simulink model "testing_embedded_matlab_functions"  (Simulink 7.5)
settings: Solver=ode45  StartTime=0.0  StopTime=10.0  RelTol=1e-3
settings Model: Creator=konstantinos  LastModifiedBy=konstantinos

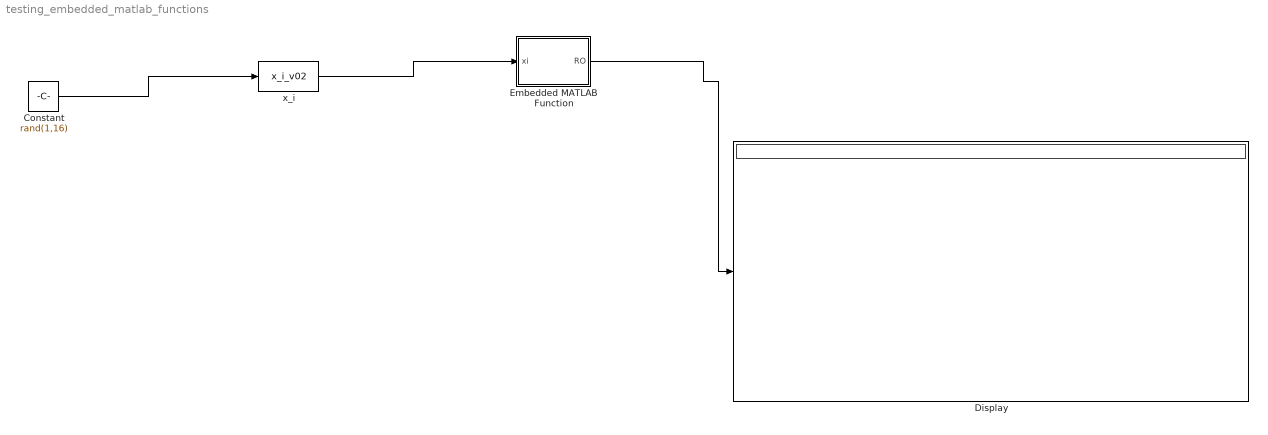
== system testing_embedded_matlab_functions ==
  Constant : Constant  Value=rand(1,16)  OutDataType=fixdt(1, 16)  OutScaling=2^0
  Display : Display
  Embedded MATLAB Function : Stateflow chart  TreatAsAtomicUnit=on
  x_i : MATLABFcn  MATLABFcn=x_i_v02  Output1D=off
  wires:
  Embedded MATLAB Function/1(RO) -> Display/1
  Constant/1 -> x_i/1
  x_i/1 -> Embedded MATLAB Function/1(xi)

== matlab function Embedded MATLAB Function ==
  data: xi input double; RO output double
%#eml
function RO=R_O(xi)



x1 = xi(1,:);
x2 = xi(2,:);
x3 = xi(3,:);
x4 = xi(4,:);

% r1=( xi(1,:)-xi(3,:) )/norm( xi(1,:)-xi(3,:) ) + ...
%     ( xi(2,:)-xi(4,:) )/norm( xi(2,:)-xi(4,:) );

r1=( x1-x3 )/norm( x1-x3 ) + ...
    ( x2-x4 )/norm( x2-x4 );


r1_unit=r1/norm(r1);

% r3= cross( (x1-x3),( x2-x4 ))';

r3= skew( x1-x3 ) * ( x2-x4 )';
r3_unit=r3/norm(r3);

r2_unit = skew(r3_unit)*r1_unit';

l=[r1_unit' r2_unit r3_unit];
RO=l;
